simulink model "SimPart2"  (R2023b)
settings: Solver=VariableStepAuto  StartTime=0.0  StopTime=2  RelTol=1e-3
settings Model: Creator=megan  LastModifiedBy=megan

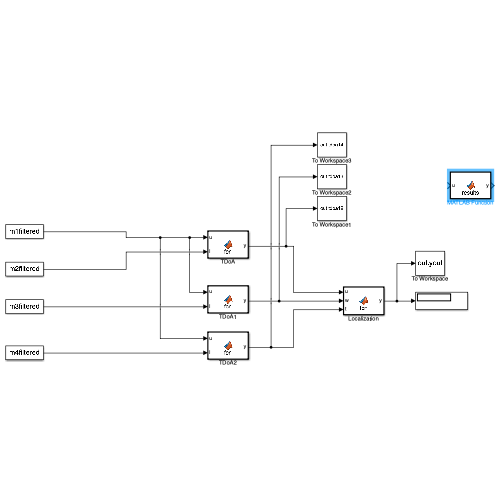
[thumbnail: Simulink's stored preview of the top-level diagram]
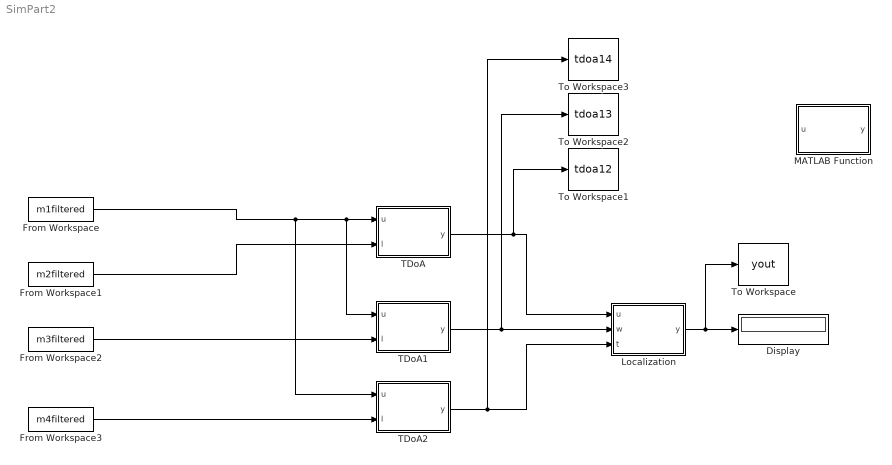
== system SimPart2 ==
  Display : Display
  From Workspace : FromWorkspace  VariableName=m1filtered
  From Workspace1 : FromWorkspace  VariableName=m2filtered
  From Workspace2 : FromWorkspace  VariableName=m3filtered
  From Workspace3 : FromWorkspace  VariableName=m4filtered
  Localization : MATLAB Function  TreatAsAtomicUnit=on
  MATLAB Function : MATLAB Function  TreatAsAtomicUnit=on
  TDoA : MATLAB Function  TreatAsAtomicUnit=on
  TDoA1 : MATLAB Function  TreatAsAtomicUnit=on
  TDoA2 : MATLAB Function  TreatAsAtomicUnit=on
  To Workspace : ToWorkspace  VariableName=yout  SampleTime=-1
      settings: Save2DSignal=2-D array (concatenate along first dimension)
  To Workspace1 : ToWorkspace  VariableName=tdoa12  SampleTime=-1
      settings: Save2DSignal=2-D array (concatenate along first dimension)
  To Workspace2 : ToWorkspace  VariableName=tdoa13  SampleTime=-1
      settings: Save2DSignal=2-D array (concatenate along first dimension)
  To Workspace3 : ToWorkspace  VariableName=tdoa14  SampleTime=-1
      settings: Save2DSignal=2-D array (concatenate along first dimension)
  wires:
  Localization/1(y) -> To Workspace/1, Display/1
  From Workspace/1 -> TDoA2/1(u), TDoA1/1(u), TDoA/1(u)
  From Workspace1/1 -> TDoA/2(l)
  From Workspace2/1 -> TDoA1/2(l)
  From Workspace3/1 -> TDoA2/2(l)
  TDoA/1(y) -> To Workspace1/1, Localization/1(u)
  TDoA1/1(y) -> To Workspace2/1, Localization/2(w)
  TDoA2/1(y) -> To Workspace3/1, Localization/3(t)

== matlab function SimPart2/Localization ==
  data: u input; y output; w input; t input
function y = fcn(u, w, t)

y = u + w + t;

== matlab function SimPart2/TDoA1 ==
  data: u input; y output; l input
function y = fcn(u, l)

y = u + l;

== matlab function SimPart2/TDoA2 ==
  data: u input; y output; l input
function y = fcn(u, l)

y = u + l;

== matlab function SimPart2/MATLAB Function ==
  data: u input; y output
function y = results(u)

%setup grid dimensions
x = 0:0.01:0.5;
y = 0:0.01:0.8;
[X Y] = meshgrid(x, y)

y = u;

== matlab function SimPart2/TDoA ==
  data: u input; y output; l input
function y = fcn(u, l)

y = u + l;
